simulink model "streamtoblock_fft"  (R2023b)
settings: Solver=FixedStepDiscrete  StartTime=0.0  StopTime=dspba_streamtosym.SimulationTime  FixedStep=1  RelTol=1e-3  EnableMultiTasking=on
PreLoadFcn:
  | setup_streamtoblock_fft;
InitFcn:
  | setup_streamtoblock_fft;
StartFcn:
  | setup_streamtoblock_fft
StopFcn:
  | %close all;
  | 
  | %plot_results;
  | 
  | %BRinput = false;
  | %BRoutput = false;
  | 
  | %analyze_subchannel_fft(...
  | %    dspb_fft_multichannel.FFTsize, ...
  | %    dspb_fft_multichannel.subchannels, ...
  | %    dspb_fft_multichannel.IFFT, ...
  | %    BRinput, BRoutput,...
  | %    v_in, chan_in, x_in,...
  | %    v_out, chan_out, z_out);
  | save('dspba_sim_op_ul.mat','Final_Dout_V','Final_Chout','Final_Dout');
  | Testanalysis
undefined symbols (not defined in the file or in its folder): dpoly, fft_tb_in_local, value
libraries: DSPBAPrim x16, simulink x15, DSPBABase x7, DSPBAModelBus x3, lib_lowphy x2
Description:
  | This design example implements a 4K-point Fast Fourier Transform.
settings Model: Creator=lrigby  LastModifiedBy=5g
settings SolverCC: AlgebraicLoopSolver=TrustRegion
settings DataIOCC: LimitDataPoints=on  SaveFormat=StructureWithTime  SignalLoggingSaveFormat=ModelDataLogs  ReturnWorkspaceOutputs=off
settings OptimizationCC: ExpressionDepthLimit=2147483647  InitFltsAndDblsToZero=on  LifeSpan=inf
settings DebuggingCC: SaveWithParameterizedLinksMsg=none  UnderspecifiedInitializationDetection=Classic  MergeDetectMultiDrivingBlocksExec=none  SignalResolutionControl=TryResolveAllWithWarning  SolverPrmCheckMsg=warning  InheritedTsInSrcMsg=none  ParameterOverflowMsg=none  ParameterPrecisionLossMsg=none  FcnCallInpInsideContextMsg=warning  UnconnectedInputMsg=warning  UnconnectedOutputMsg=warning  UnconnectedLineMsg=warning  StateNameClashWarn=warning  SFUnexpectedBacktrackingDiag=warning  SFNoUnconditionalDefaultTransitionDiag=warning  ArithmeticOperatorsInVariantConditions=warning
settings HardwareCC: ProdBitPerPointer=32  ProdBitPerSizeT=32  ProdBitPerPtrDiffT=32  ProdLargestAtomicFloat=None  ProdIntDivRoundTo=Undefined  ProdEndianess=Unspecified  ProdWordSize=32  ProdHWDeviceType=ASIC/FPGA  TargetBitPerLong=64  TargetBitPerPointer=64  TargetBitPerSizeT=64  TargetBitPerPtrDiffT=64  TargetLongLongMode=on  TargetIntDivRoundTo=Zero  TargetEndianess=LittleEndian  TargetWordSize=64  TargetHWDeviceType=MATLAB Host  ProdEqTarget=off
settings ModelReferenceCC: EnableRefExpFcnMdlSchedulingChecks=on  PropagateSignalLabelsOutOfModel=off
settings SFSimCC: SimUseLocalCustomCode=off  SimParseCustomCode=off  CustomCodeUndefinedFunction=UseInterfaceOnly
settings RTWCC: RTWUseLocalCustomCode=off  DLArmComputeVersion=19.05
settings CodeAppCC: StateflowObjectComments=on
settings GRTTargetCC: TargetFcnLib=ansi_tfl_tmw.mat  TargetLangStandard=C89/C90 (ANSI)  CombineOutputUpdateFcns=off  GRTInterface=on
settings ConfigComp: CovMetricSettings=dw  CovSaveCumulativeToWorkspaceVar=on  CovSaveSingleToWorkspaceVar=on  CovExternalEMLEnable=off  CovSFcnEnable=off

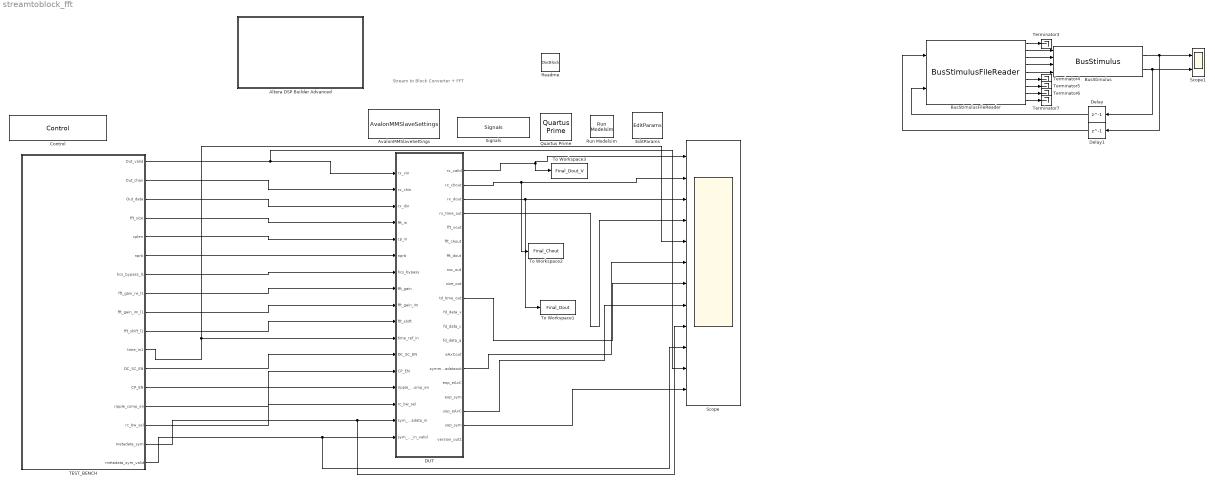
== system streamtoblock_fft ==
  note: Stream to Block Converter + FFT
  Altera DSP Builder Advanced : Subsystem  mask(DSP Builder Advanced Blockset Ignored Block){}
      settings: OpenFcn=web('http://www.altera.com', '-new');
      mask Display: image(imread('alteralogo.tif'));
  AvalonMMSlaveSettings : DSPBABase/AvalonMMSlaveSettings
  BusStimulus : DSPBAModelBus/BusStimulus  SampleTime=1  version=20140122  hasreaden=on
  BusStimulusFileReader : DSPBAModelBus/BusStimulusFileReader  enabled=on  filename=demo_regs_stimuli.stm  logfilename=demo_regs_stimuli.log  spacewidth=2  addrwidth=14  datawidth=32  SampleTime=-1  version=20140124  hasreaden=on
  Control : DSPBABase/Control  generate=on  language=VHDL  destination=rtl  make_full_path=off  path_is_relative=on  autotestbench=on  signaldepth=2  coveragetestbench=off  logs=off  spacewidth=2  spacenum=1  addrwidth=10  datawidth=16  dataendian=Big Endian  hierarchicalnames=on  ramThresholdBits=-1  distRamThresholdBits=-1  mlabThresholdBits=-1  hardMultiplierThresholdLuts=-1  version=20090407  errorOnChanMismatch=1  errorOnGPIOMismatch=0  importModelsimResults=0  cycleAccurate=off  reinterpretCastMult=off  paramFile=streamtoblock_fft_params.xml
  DUT : Subsystem
  Delay : Delay  DelayLength=1
  Delay1 : Delay  DelayLength=1
  EditParams : DSPBABase/EditParams  version=20090407
  Quartus Prime : DSPBABase/Quartus Prime  version=20090407
  Readme : simulink/Model-Wide Utilities/DocBlock  DocumentType=Text
      content=|
      | Model version : 1.0
      | Date : 28-06-2023
      |
      | This model contains simulation of low phy system for 5G NR . This includes stream to blick conversion, CP removal, Rx gain, Phase compensation etc
      |
      |
      | Steps to run this model.
      | 1. Different test cases are noted in datagen_testcase_Run.m file
      | 2. Depending on the test case selection , input -output test vectors are stored in test_case_file.mat.
      | 3. Test bench in the .mdl file is loaded from contents of test_case_file.mat.
      | 4. Model is run automatically and then test analysis is run to check for errors.
  Run Modelsim : DSPBABase/Run Modelsim  version=20090407
  Scope : Scope  NumInputPorts=12
  Scope1 : Scope  NumInputPorts=2
  Signals : DSPBABase/Signals  clk=clk  freq=240  margin=0  rst=areset  rstactive=High  bus=bus  enbusclock=off  busfreq=491.52  bussync=off  version=20090407
  TEST_BENCH : Subsystem
  Terminator{3..7} (5 alike) : Terminator
  To Workspace1 : ToWorkspace  VariableName=Final_Dout  SaveFormat=Timeseries  SampleTime=-1
  To Workspace2 : ToWorkspace  VariableName=Final_Chout  SaveFormat=Timeseries  SampleTime=-1
  To Workspace3 : ToWorkspace  VariableName=Final_Dout_V  SaveFormat=Timeseries  SampleTime=-1
  wires:
  TEST_BENCH/1(Out_valid) -> Scope/11, DUT/1(rx_vin)
  TEST_BENCH/2(Out_chan) -> DUT/2(rx_chin)
  TEST_BENCH/3(Out_data) -> DUT/3(rx_din)
  TEST_BENCH/4(fft_size) -> DUT/4(fft_in)
  TEST_BENCH/5(cplen) -> DUT/5(cp_in)
  TEST_BENCH/6(nprb) -> DUT/6(nprb)
  TEST_BENCH/7(hcs_bypass_l1) -> DUT/7(hcs_bypass)
  TEST_BENCH/8(fft_gain_re_l1) -> DUT/8(fft_gain)
  TEST_BENCH/9(fft_gain_im_l1) -> DUT/9(fft_gain_im)
  TEST_BENCH/10(fft_shift_l1) -> DUT/10(fft_shift)
  TEST_BENCH/11(time_in1) -> Scope/5, DUT/11(time_ref_in)
  TEST_BENCH/12(DC_SC_EN) -> DUT/12(DC_SC_EN)
  DUT/4(rx_time_out) -> Scope/4
  DUT/3(rx_dout) -> To Workspace1/1, Scope/3
  DUT/2(rx_chout) -> To Workspace2/1, Scope/2
  DUT/1(rx_valid) -> To Workspace3/1, Scope/1
  TEST_BENCH/13(CP_EN) -> DUT/13(CP_EN)
  BusStimulusFileReader/8 -> Terminator6/1
  BusStimulusFileReader/1 -> Terminator3/1
  BusStimulusFileReader/3 -> BusStimulus/2
  Delay1/1 -> BusStimulusFileReader/1
  BusStimulusFileReader/6 -> Terminator4/1
  BusStimulusFileReader/7 -> Terminator5/1
  BusStimulus/2 -> Delay/1, Scope1/2
  BusStimulusFileReader/5 -> BusStimulus/4
  Delay/1 -> BusStimulusFileReader/2
  BusStimulus/1 -> Delay1/1, Scope1/1
  BusStimulusFileReader/4 -> BusStimulus/3
  BusStimulusFileReader/2 -> BusStimulus/1
  BusStimulusFileReader/9 -> Terminator7/1
  TEST_BENCH/14(ripple_comp_en) -> DUT/14(ripple_comp_en)
  TEST_BENCH/15(rc_bw_sel) -> DUT/15(rc_bw_sel)
  TEST_BENCH/16(metadata_sym) -> Scope/9, DUT/16(sym_metadata_in)
  TEST_BENCH/17(metadata_sym_valid) -> Scope/10, DUT/17(sym_metadata_in_valid)
  DUT/15(symmetadataout) -> Scope/6
  DUT/10(td_time_out) -> Scope/7
  DUT/18(sop_eAxC) -> Scope/8
  DUT/19(sop_sym) -> Scope/12

== system streamtoblock_fft/Altera DSP Builder Advanced ==

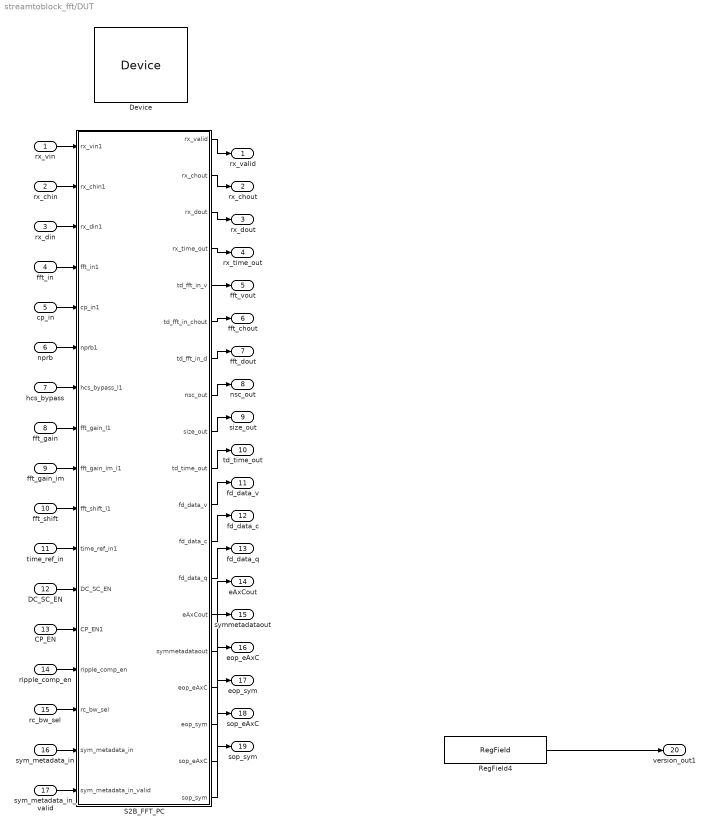
== system streamtoblock_fft/DUT ==
  rx_vin : Inport
  rx_chin : Inport  Port=2
  rx_din : Inport  Port=3
  fft_in : Inport  Port=4
  cp_in : Inport  Port=5
  nprb : Inport  Port=6
  hcs_bypass : Inport  Port=7
  fft_gain : Inport  Port=8
  fft_gain_im : Inport  Port=9
  fft_shift : Inport  Port=10
  time_ref_in : Inport  Port=11
  DC_SC_EN : Inport  Port=12
  CP_EN : Inport  Port=13
  ripple_comp_en : Inport  Port=14
  rc_bw_sel : Inport  Port=15
  sym_metadata_in : Inport  Port=16
  sym_metadata_in_valid : Inport  Port=17
  Device : DSPBABase/Device  family=Arria 10  stratix4device=Stratix IV E  hardcopy4device=HardCopy IV E  stratix5device=Stratix V GX  device=AUTO  speed=1  stratixSpeed=-5  stratix2Speed=-3  stratix3Speed=-2  stratix4gxSpeed=-2  stratix4gtSpeed=-1  cyclone2Speed=-6  cyclone3Speed=-7  arria2Speed=-4  cyclone4eSpeed=-8  stratix5Speed=-3  arria5Speed=-4  arriaSpeed=-6  cyclone3lsSpeed=-7  cyclone5Speed=-6  arria2gzSpeed=-3  nightFurySpeed=-2  ecp2Speed=-7  hardcopycompat=off  version=20140217  max10flashmode=off  max10nomeminit=off
  RegField4 : DSPBAModelBus/RegField  reg_name=reg_mem_offset_version  reg_rwmode=Read/Write  reg_msb=31  reg_lsb=0  reg_mode=Specify via dialog  reg_type=ufix(32)  reg_scale=2^0  reg_init=Version_reg_val  reg_desc=version_out  reg_modal=off  reg_desc0=0  reg_desc1=0  reg_desc2=0  reg_desc3=0  reg_desc4=0  reg_desc5=0  reg_desc6=0  reg_desc7=0  reg_addr=7  SampleTime=-1  version=20090407
  S2B_FFT_PC : Subsystem
  rx_valid : Outport
  rx_chout : Outport  Port=2
  rx_dout : Outport  Port=3
  rx_time_out : Outport  Port=4
  fft_vout : Outport  Port=5
  fft_chout : Outport  Port=6
  fft_dout : Outport  Port=7
  nsc_out : Outport  Port=8
  size_out : Outport  Port=9
  td_time_out : Outport  Port=10
  fd_data_v : Outport  Port=11
  fd_data_c : Outport  Port=12
  fd_data_q : Outport  Port=13
  eAxCout : Outport  Port=14
  symmetadataout : Outport  Port=15
  eop_eAxC : Outport  Port=16
  eop_sym : Outport  Port=17
  sop_eAxC : Outport  Port=18
  sop_sym : Outport  Port=19
  version_out1 : Outport  Port=20
  wires:
  S2B_FFT_PC/19(sop_sym) -> sop_sym/1
  S2B_FFT_PC/16(eop_eAxC) -> eop_eAxC/1
  S2B_FFT_PC/14(eAxCout) -> eAxCout/1
  CP_EN/1 -> S2B_FFT_PC/13(CP_EN1)
  fft_gain_im/1 -> S2B_FFT_PC/9(fft_gain_im_l1)
  S2B_FFT_PC/15(symmetadataout) -> symmetadataout/1
  fft_in/1 -> S2B_FFT_PC/4(fft_in1)
  DC_SC_EN/1 -> S2B_FFT_PC/12(DC_SC_EN)
  S2B_FFT_PC/13(fd_data_q) -> fd_data_q/1
  fft_shift/1 -> S2B_FFT_PC/10(fft_shift_l1)
  rx_vin/1 -> S2B_FFT_PC/1(rx_vin1)
  cp_in/1 -> S2B_FFT_PC/5(cp_in1)
  rx_chin/1 -> S2B_FFT_PC/2(rx_chin1)
  S2B_FFT_PC/12(fd_data_c) -> fd_data_c/1
  hcs_bypass/1 -> S2B_FFT_PC/7(hcs_bypass_l1)
  time_ref_in/1 -> S2B_FFT_PC/11(time_ref_in1)
  rc_bw_sel/1 -> S2B_FFT_PC/15(rc_bw_sel)
  S2B_FFT_PC/1(rx_valid) -> rx_valid/1
  sym_metadata_in/1 -> S2B_FFT_PC/16(sym_metadata_in)
  sym_metadata_in_valid/1 -> S2B_FFT_PC/17(sym_metadata_in_valid)
  nprb/1 -> S2B_FFT_PC/6(nprb1)
  S2B_FFT_PC/2(rx_chout) -> rx_chout/1
  S2B_FFT_PC/6(td_fft_in_chout) -> fft_chout/1
  S2B_FFT_PC/4(rx_time_out) -> rx_time_out/1
  S2B_FFT_PC/17(eop_sym) -> eop_sym/1
  rx_din/1 -> S2B_FFT_PC/3(rx_din1)
  S2B_FFT_PC/3(rx_dout) -> rx_dout/1
  S2B_FFT_PC/7(td_fft_in_d) -> fft_dout/1
  S2B_FFT_PC/5(td_fft_in_v) -> fft_vout/1
  S2B_FFT_PC/8(nsc_out) -> nsc_out/1
  S2B_FFT_PC/9(size_out) -> size_out/1
  fft_gain/1 -> S2B_FFT_PC/8(fft_gain_l1)
  S2B_FFT_PC/10(td_time_out) -> td_time_out/1
  S2B_FFT_PC/18(sop_eAxC) -> sop_eAxC/1
  ripple_comp_en/1 -> S2B_FFT_PC/14(ripple_comp_en)
  S2B_FFT_PC/11(fd_data_v) -> fd_data_v/1
  RegField4/1 -> version_out1/1

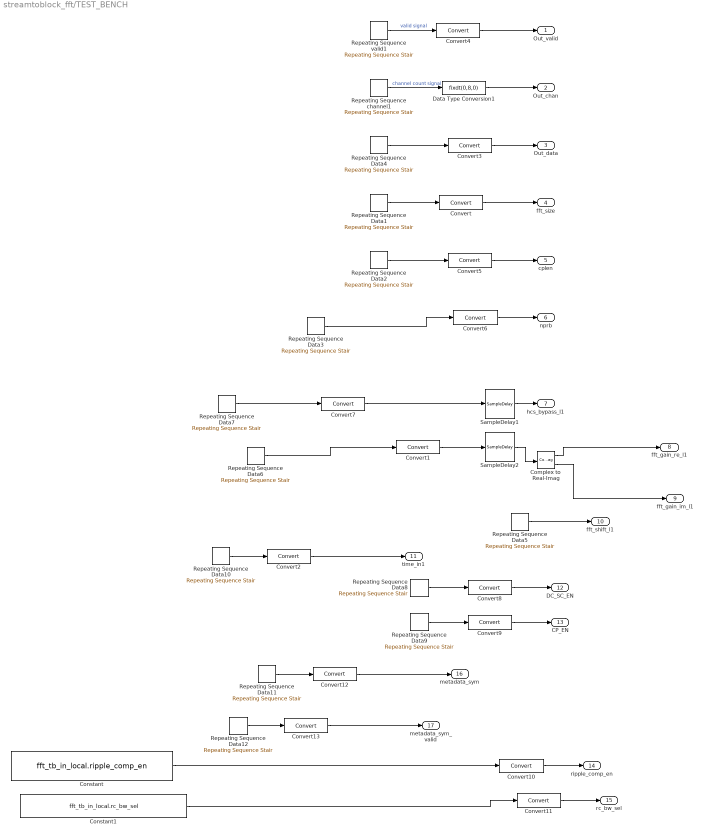
== system streamtoblock_fft/TEST_BENCH ==
  Complex to Real-Imag : ComplexToRealImag
  Constant : Constant  Value=fft_tb_in_local.ripple_comp_en  SampleTime=1
  Constant1 : Constant  Value=fft_tb_in_local.rc_bw_sel  SampleTime=1
  Convert : DSPBAPrim/Convert  primtype=convert  nInputs=1  nOutputs=1  omode=Specify via dialog  otype=ufix(4)  scale=2^0  rndmethod=Biased  factor=1  satmethod=None  shift_vec=[0 1 2 -1]  value=round([0:255]/17)  inPortNames=[' '; ' ';]  outPortNames=[' '; 'c']  dspbaimage=dspba_prim_wide.svg  text=fprintf('convert');  style=Optimised  visibilities=8+64+256+2^17  clipdetect=off  floatPrecision=float32_m23  advOptions=[]  version=20211007
  Convert1 : DSPBAPrim/Convert  primtype=convert  nInputs=1  nOutputs=1  omode=Specify via dialog  otype=fixdt(0,16,14)  scale=0  rndmethod=Biased  factor=1  satmethod=Symmetric  shift_vec=[0 1 2 -1]  value=round([0:255]/17)  inPortNames=[' '; ' ';]  outPortNames=[' '; 'c']  dspbaimage=dspba_prim_wide.svg  text=fprintf('convert');  style=Optimised  visibilities=8+64+256+2^17  clipdetect=off  floatPrecision=float32_m23  advOptions=[]  version=20211007
  Convert{8..11} (4 alike) : DSPBAPrim/Convert  primtype=convert  nInputs=1  nOutputs=1  omode=boolean  otype=fixdt(0,12,0)  scale=0  rndmethod=Biased  factor=1  satmethod=None  shift_vec=[0 1 2 -1]  value=round([0:255]/17)  inPortNames=[' '; ' ';]  outPortNames=[' '; 'c']  dspbaimage=dspba_prim_wide.svg  text=fprintf('convert');  style=Optimised  visibilities=8+64+256+2^17  clipdetect=off  floatPrecision=float32_m23  advOptions=[]  version=20211007
  Convert12 : DSPBAPrim/Convert  primtype=convert  nInputs=1  nOutputs=1  omode=Specify via dialog  otype=ufix(64)  scale=2^0  rndmethod=Biased  factor=1  satmethod=None  shift_vec=[0 1 2 -1]  value=round([0:255]/17)  inPortNames=[' '; ' ';]  outPortNames=[' '; 'c']  dspbaimage=dspba_prim_wide.svg  text=fprintf('convert');  style=Optimised  visibilities=8+64+256+2^17  clipdetect=off  floatPrecision=float32_m23  advOptions=[]  version=20211007
  Convert13 : DSPBAPrim/Convert  primtype=convert  nInputs=1  nOutputs=1  omode=boolean  otype=ufix(64)  scale=2^0  rndmethod=Biased  factor=1  satmethod=None  shift_vec=[0 1 2 -1]  value=round([0:255]/17)  inPortNames=[' '; ' ';]  outPortNames=[' '; 'c']  dspbaimage=dspba_prim_wide.svg  text=fprintf('convert');  style=Optimised  visibilities=8+64+256+2^17  clipdetect=off  floatPrecision=float32_m23  advOptions=[]  version=20211007
  Convert2 : DSPBAPrim/Convert  primtype=convert  nInputs=1  nOutputs=1  omode=Specify via dialog  otype=ufix(64)  scale=2^0  rndmethod=Biased  factor=1  satmethod=None  shift_vec=[0 1 2 -1]  value=round([0:255]/17)  inPortNames=[' '; ' ';]  outPortNames=[' '; 'c']  dspbaimage=dspba_prim_wide.svg  text=fprintf('convert');  style=Optimised  visibilities=8+64+256+2^17  clipdetect=off  floatPrecision=float32_m23  advOptions=[]  version=20211007
  Convert3 : DSPBAPrim/Convert  primtype=convert  nInputs=1  nOutputs=1  omode=Specify via dialog  otype=fixdt(1,16,14)  scale=0  rndmethod=Biased  factor=1  satmethod=None  shift_vec=[0 1 2 -1]  value=round([0:255]/17)  inPortNames=[' '; ' ';]  outPortNames=[' '; 'c']  dspbaimage=dspba_prim_wide.svg  text=fprintf('convert');  style=Optimised  visibilities=8+64+256+2^17  clipdetect=off  floatPrecision=float32_m23  advOptions=[]  version=20211007
  Convert4 : DSPBAPrim/Convert  primtype=convert  nInputs=1  nOutputs=1  omode=boolean  otype=ufix(4)  scale=2^0  rndmethod=Biased  factor=1  satmethod=None  shift_vec=[0 1 2 -1]  value=round([0:255]/17)  inPortNames=[' '; ' ';]  outPortNames=[' '; 'c']  dspbaimage=dspba_prim_wide.svg  text=fprintf('convert');  style=Optimised  visibilities=8+64+256+2^17  clipdetect=off  floatPrecision=float32_m23  advOptions=[]  version=20211007
  Convert5 : DSPBAPrim/Convert  primtype=convert  nInputs=1  nOutputs=1  omode=Specify via dialog  otype=fixdt(0,16,0)  scale=0  rndmethod=Biased  factor=1  satmethod=None  shift_vec=[0 1 2 -1]  value=round([0:255]/17)  inPortNames=[' '; ' ';]  outPortNames=[' '; 'c']  dspbaimage=dspba_prim_wide.svg  text=fprintf('convert');  style=Optimised  visibilities=8+64+256+2^17  clipdetect=off  floatPrecision=float32_m23  advOptions=[]  version=20211007
  Convert6 : DSPBAPrim/Convert  primtype=convert  nInputs=1  nOutputs=1  omode=Specify via dialog  otype=fixdt(0,16,0)  scale=0  rndmethod=Biased  factor=1  satmethod=None  shift_vec=[0 1 2 -1]  value=round([0:255]/17)  inPortNames=[' '; ' ';]  outPortNames=[' '; 'c']  dspbaimage=dspba_prim_wide.svg  text=fprintf('convert');  style=Optimised  visibilities=8+64+256+2^17  clipdetect=off  floatPrecision=float32_m23  advOptions=[]  version=20211007
  Convert7 : DSPBAPrim/Convert  primtype=convert  nInputs=1  nOutputs=1  omode=boolean  otype=sfix(16)  scale=2^-15  rndmethod=Biased  factor=1  satmethod=Symmetric  shift_vec=[0 1 2 -1]  value=round([0:255]/17)  inPortNames=[' '; ' ';]  outPortNames=[' '; 'c']  dspbaimage=dspba_prim_wide.svg  text=fprintf('convert');  style=Optimised  visibilities=8+64+256+2^17  clipdetect=off  floatPrecision=float32_m23  advOptions=[]  version=20211007
  Data Type Conversion1 : DataTypeConversion  OutDataTypeStr=fixdt(0,8,0)  SaturateOnIntegerOverflow=off  RndMeth=Floor
  Repeating Sequence Data1 : simulink/Sources/Repeating Sequence Stair  OutValues=fft_tb_in_local.fftsize_in  tsamp=1  OutMin=[]  OutMax=[]  OutDataTypeStr=uint16  OutputDataTypeScalingMode=uint16  OutDataType=fixdt(0,8)  ConRadixGroup=Best Precision: Vector-wise  OutScaling=2^-12
  Repeating Sequence Data10 : simulink/Sources/Repeating Sequence Stair  OutValues=fft_tb_in_local.Tsym  tsamp=1  OutMin=[]  OutMax=[]  OutDataTypeStr=double  OutputDataTypeScalingMode=double  OutDataType=fixdt(1,16,15)  ConRadixGroup=Best Precision: Vector-wise  OutScaling=[]
  Repeating Sequence Data11 : simulink/Sources/Repeating Sequence Stair  OutValues=fft_tb_in_local.metadata_sym  tsamp=1  OutMin=[]  OutMax=[]  OutDataTypeStr=double  OutputDataTypeScalingMode=double  OutDataType=fixdt(1,16,15)  ConRadixGroup=Best Precision: Vector-wise  OutScaling=[]
  Repeating Sequence Data12 : simulink/Sources/Repeating Sequence Stair  OutValues=fft_tb_in_local.metadata_sym_valid  tsamp=1  OutMin=[]  OutMax=[]  OutDataTypeStr=double  OutputDataTypeScalingMode=double  OutDataType=fixdt(1,16,15)  ConRadixGroup=Best Precision: Vector-wise  OutScaling=[]
  Repeating Sequence Data2 : simulink/Sources/Repeating Sequence Stair  OutValues=fft_tb_in_local.CPLen_in  tsamp=1  OutMin=[]  OutMax=[]  OutDataTypeStr=uint16  OutputDataTypeScalingMode=uint16  OutDataType=fixdt(1,16,15)  ConRadixGroup=Best Precision: Vector-wise  OutScaling=[]
  Repeating Sequence Data3 : simulink/Sources/Repeating Sequence Stair  OutValues=fft_tb_in_local.nprb_v  tsamp=1  OutMin=[]  OutMax=[]  OutDataTypeStr=double  OutputDataTypeScalingMode=double  OutDataType=fixdt(1,16,15)  ConRadixGroup=Best Precision: Vector-wise  OutScaling=[]
  Repeating Sequence Data4 : simulink/Sources/Repeating Sequence Stair  OutValues=fft_tb_in_local.dout_v  tsamp=1  OutMin=[]  OutMax=[]  OutDataTypeStr=fixdt(1,16,14)  OutputDataTypeScalingMode=Specify via dialog  OutDataType=fixdt(1,16,14)  ConRadixGroup=Best Precision: Vector-wise  OutScaling=[]
  Repeating Sequence Data5 : simulink/Sources/Repeating Sequence Stair  OutValues=fft_tb_in_local.ifftshift_v  tsamp=1  OutMin=[]  OutMax=[]  OutDataTypeStr=fixdt(0,4,0)  OutputDataTypeScalingMode=Specify via dialog  OutDataType=fixdt(0,4,0)  ConRadixGroup=Best Precision: Vector-wise  OutScaling=[]
  Repeating Sequence Data6 : simulink/Sources/Repeating Sequence Stair  OutValues=fft_tb_in_local.const_gain_v  tsamp=1  OutMin=[]  OutMax=[]  OutDataTypeStr=double  OutputDataTypeScalingMode=double  OutDataType=fixdt(1,16,15)  ConRadixGroup=Best Precision: Vector-wise  OutScaling=[]
  Repeating Sequence Data7 : simulink/Sources/Repeating Sequence Stair  OutValues=fft_tb_in_local.hcshift_v  tsamp=1  OutMin=[]  OutMax=[]  OutDataTypeStr=double  OutputDataTypeScalingMode=double  OutDataType=fixdt(1,16,15)  ConRadixGroup=Best Precision: Vector-wise  OutScaling=[]
  Repeating Sequence Data8 : simulink/Sources/Repeating Sequence Stair  OutValues=fft_tb_in_local.DC_SC_EN  tsamp=1  OutMin=[]  OutMax=[]  OutDataTypeStr=double  OutputDataTypeScalingMode=double  OutDataType=fixdt(1,16,15)  ConRadixGroup=Best Precision: Vector-wise  OutScaling=[]
  Repeating Sequence Data9 : simulink/Sources/Repeating Sequence Stair  OutValues=fft_tb_in_local.Tech_CP  tsamp=1  OutMin=[]  OutMax=[]  OutDataTypeStr=double  OutputDataTypeScalingMode=double  OutDataType=fixdt(1,16,15)  ConRadixGroup=Best Precision: Vector-wise  OutScaling=[]
  Repeating Sequence channel1 : simulink/Sources/Repeating Sequence Stair  OutValues=fft_tb_in_local.chout_v  tsamp=1  OutMin=[]  OutMax=[]  OutDataTypeStr=uint8  OutputDataTypeScalingMode=uint8  OutDataType=fixdt(1,16)  ConRadixGroup=Best Precision: Vector-wise  OutScaling=[]
  Repeating Sequence valid1 : simulink/Sources/Repeating Sequence Stair  OutValues=fft_tb_in_local.valid_out  tsamp=1  OutMin=[]  OutMax=[]  OutDataTypeStr=fixdt('boolean')  OutputDataTypeScalingMode=Specify via dialog  OutDataType=fixdt('boolean')  ConRadixGroup=Best Precision: Vector-wise  OutScaling=[]
  SampleDelay1 : DSPBAPrim/SampleDelay  primtype=sampdelay  nInputs=1  nOutputs=1  omode=Inherit via internal rule  otype=sfix(16)  scale=2^-15  rndmethod=Unbiased  factor=1  satmethod=Symmetric  shift_vec=[0 1 2 -1]  floatPrecision=float32_m23  value=100  inPortNames=[' '; ' ';]  outPortNames=[' ']  dspbaimage=dspba_prim.svg  text=dpoly(1, eye(1,value+1), 'z')  style=Optimised  visibilities=8 + 1024 + 2^17 + 2^18  flexible=off  slackgroup=0  augmented=0  version=20211007  advOptions=[]
  SampleDelay2 : DSPBAPrim/SampleDelay  primtype=sampdelay  nInputs=1  nOutputs=1  omode=Inherit via internal rule  otype=sfix(16)  scale=2^-15  rndmethod=Unbiased  factor=1  satmethod=Symmetric  shift_vec=[0 1 2 -1]  floatPrecision=float32_m23  value=100  inPortNames=[' '; ' ';]  outPortNames=[' ']  dspbaimage=dspba_prim.svg  text=dpoly(1, eye(1,value+1), 'z')  style=Optimised  visibilities=8 + 1024 + 2^17 + 2^18  flexible=off  slackgroup=0  augmented=0  version=20211007  advOptions=[]
  Out_valid : Outport
  Out_chan : Outport  Port=2
  Out_data : Outport  Port=3
  fft_size : Outport  Port=4
  cplen : Outport  Port=5
  nprb : Outport  Port=6
  hcs_bypass_l1 : Outport  Port=7
  fft_gain_re_l1 : Outport  Port=8
  fft_gain_im_l1 : Outport  Port=9
  fft_shift_l1 : Outport  Port=10
  time_in1 : Outport  Port=11
  DC_SC_EN : Outport  Port=12
  CP_EN : Outport  Port=13
  ripple_comp_en : Outport  Port=14
  rc_bw_sel : Outport  Port=15
  metadata_sym : Outport  Port=16
  metadata_sym_valid : Outport  Port=17
  wires:
  Repeating Sequence channel1/1 -> Data Type Conversion1/1  "channel count signal"
  Repeating Sequence valid1/1 -> Convert4/1  "valid signal"
  Repeating Sequence Data4/1 -> Convert3/1
  Repeating Sequence Data1/1 -> Convert/1
  Repeating Sequence Data2/1 -> Convert5/1
  Data Type Conversion1/1 -> Out_chan/1
  Convert/1 -> fft_size/1
  Repeating Sequence Data7/1 -> Convert7/1
  Convert7/1 -> SampleDelay1/1
  Convert1/1 -> SampleDelay2/1
  SampleDelay1/1 -> hcs_bypass_l1/1
  Repeating Sequence Data5/1 -> fft_shift_l1/1
  Convert2/1 -> time_in1/1
  Convert3/1 -> Out_data/1
  Convert4/1 -> Out_valid/1
  Convert5/1 -> cplen/1
  Convert6/1 -> nprb/1
  Repeating Sequence Data3/1 -> Convert6/1
  SampleDelay2/1 -> Complex to Real-Imag/1
  Complex to Real-Imag/1 -> fft_gain_re_l1/1
  Complex to Real-Imag/2 -> fft_gain_im_l1/1
  Repeating Sequence Data6/1 -> Convert1/1
  Repeating Sequence Data8/1 -> Convert8/1
  Convert8/1 -> DC_SC_EN/1
  Convert9/1 -> CP_EN/1
  Repeating Sequence Data9/1 -> Convert9/1
  Repeating Sequence Data10/1 -> Convert2/1
  Convert10/1 -> ripple_comp_en/1
  Constant/1 -> Convert10/1
  Constant1/1 -> Convert11/1
  Convert11/1 -> rc_bw_sel/1
  Convert12/1 -> metadata_sym/1
  Repeating Sequence Data11/1 -> Convert12/1
  Repeating Sequence Data12/1 -> Convert13/1
  Convert13/1 -> metadata_sym_valid/1

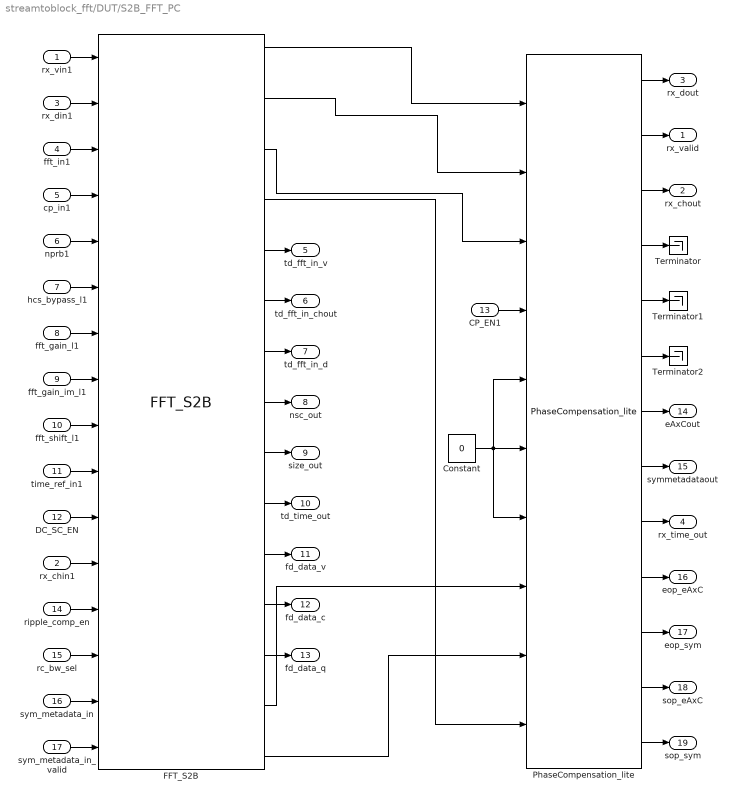
== system streamtoblock_fft/DUT/S2B_FFT_PC ==
  rx_vin1 : Inport
  rx_chin1 : Inport  Port=2
  rx_din1 : Inport  Port=3
  fft_in1 : Inport  Port=4
  cp_in1 : Inport  Port=5
  nprb1 : Inport  Port=6
  hcs_bypass_l1 : Inport  Port=7
  fft_gain_l1 : Inport  Port=8
  fft_gain_im_l1 : Inport  Port=9
  fft_shift_l1 : Inport  Port=10
  time_ref_in1 : Inport  Port=11
  DC_SC_EN : Inport  Port=12
  CP_EN1 : Inport  Port=13
  ripple_comp_en : Inport  Port=14
  rc_bw_sel : Inport  Port=15
  sym_metadata_in : Inport  Port=16
  sym_metadata_in_valid : Inport  Port=17
  Constant : Constant  Value=0
  FFT_S2B : lib_lowphy/FFT_S2B  FFTmaxsize=12  FFTminsize=9  FFTstages=12  Rx_scaling=2^-12  AxCdelay=288  NCO_addr_offset=9  rc_out_frac=11
      link override CPRemoval/ChannelOut: latency=10
      link override CPRemoval/Mem_rd_sub1/SampleDelay2: augmented=0
      link override SignalProcessing/BRandSCSelect1/channel_BRSC1_in: dataSignals=9
      link override SignalProcessing/BRandSCSelect1/channel_BRSC1_out: dataSignals=5  latency=17
      link override SignalProcessing/HCShift/NCO: latency=14
      link override SignalProcessing/HCShift/Subsystem/channel_HSC1_out: latency=0
      link override SignalProcessing/RXGainComp/channel_RXG1_out: latency=7
      link override SignalProcessing/RXScaling/channel_RXS1_out: latency=4
      link override SignalProcessing/VFFT_btb/channel_FFT1_out: latency=68
  PhaseCompensation_lite : lib_lowphy/PhaseCompensation_lite  Tc=1/122.88e6  CP_1=352  CP_2=288  PhaseGen_TXRX=0  Op_frac_scaling=2^-11  reg_mem_offset_rf_freq=4  reg_mem_offset_Phase_comp_enable=5  reg_mem_offset_tx_rx_sel=6
      link override ComplexMixer/ComplexMixer: latency=5
      link override SOP_EOP_gen/channel_RXG1_out: latency=0
  Terminator : Terminator
  Terminator1 : Terminator
  Terminator2 : Terminator
  rx_valid : Outport
  rx_chout : Outport  Port=2
  rx_dout : Outport  Port=3
  rx_time_out : Outport  Port=4
  td_fft_in_v : Outport  Port=5
  td_fft_in_chout : Outport  Port=6
  td_fft_in_d : Outport  Port=7
  nsc_out : Outport  Port=8
  size_out : Outport  Port=9
  td_time_out : Outport  Port=10
  fd_data_v : Outport  Port=11
  fd_data_c : Outport  Port=12
  fd_data_q : Outport  Port=13
  eAxCout : Outport  Port=14
  symmetadataout : Outport  Port=15
  eop_eAxC : Outport  Port=16
  eop_sym : Outport  Port=17
  sop_eAxC : Outport  Port=18
  sop_sym : Outport  Port=19
  wires:
  PhaseCompensation_lite/6 -> Terminator2/1
  PhaseCompensation_lite/4 -> Terminator/1
  PhaseCompensation_lite/3 -> rx_chout/1
  FFT_S2B/13 -> fd_data_q/1
  time_ref_in1/1 -> FFT_S2B/10
  PhaseCompensation_lite/1 -> rx_dout/1
  CP_EN1/1 -> PhaseCompensation_lite/4
  fft_gain_im_l1/1 -> FFT_S2B/8
  rx_vin1/1 -> FFT_S2B/1
  nprb1/1 -> FFT_S2B/5
  fft_in1/1 -> FFT_S2B/3
  fft_shift_l1/1 -> FFT_S2B/9
  cp_in1/1 -> FFT_S2B/4
  ripple_comp_en/1 -> FFT_S2B/13
  PhaseCompensation_lite/5 -> Terminator1/1
  rx_din1/1 -> FFT_S2B/2
  fft_gain_l1/1 -> FFT_S2B/7
  FFT_S2B/6 -> td_fft_in_chout/1
  rx_chin1/1 -> FFT_S2B/12
  FFT_S2B/3 -> PhaseCompensation_lite/3
  DC_SC_EN/1 -> FFT_S2B/11
  rc_bw_sel/1 -> FFT_S2B/14
  FFT_S2B/10 -> td_time_out/1
  FFT_S2B/1 -> PhaseCompensation_lite/1
  PhaseCompensation_lite/2 -> rx_valid/1
  FFT_S2B/2 -> PhaseCompensation_lite/2
  FFT_S2B/11 -> fd_data_v/1
  FFT_S2B/5 -> td_fft_in_v/1
  FFT_S2B/7 -> td_fft_in_d/1
  FFT_S2B/8 -> nsc_out/1
  Constant/1 -> PhaseCompensation_lite/5, PhaseCompensation_lite/7, PhaseCompensation_lite/6
  FFT_S2B/9 -> size_out/1
  hcs_bypass_l1/1 -> FFT_S2B/6
  FFT_S2B/12 -> fd_data_c/1
  FFT_S2B/14 -> PhaseCompensation_lite/8
  FFT_S2B/4 -> PhaseCompensation_lite/10
  FFT_S2B/15 -> PhaseCompensation_lite/9
  PhaseCompensation_lite/9 -> rx_time_out/1
  PhaseCompensation_lite/7 -> eAxCout/1
  PhaseCompensation_lite/8 -> symmetadataout/1
  PhaseCompensation_lite/10 -> eop_eAxC/1
  PhaseCompensation_lite/11 -> eop_sym/1
  PhaseCompensation_lite/12 -> sop_eAxC/1
  PhaseCompensation_lite/13 -> sop_sym/1
  sym_metadata_in/1 -> FFT_S2B/15
  sym_metadata_in_valid/1 -> FFT_S2B/16
